simulink model "GP_CTC"  (R2019a)
settings: Solver=FixedStepAuto  StartTime=0  StopTime=300  FixedStep=0.005  RelTol=1e-3
model workspace: external: MAT-File (data not in the file)
libraries: RealTimeLearning x2, simulink x1
settings Model: SnapshotBufferSize=1  SnapshotInterval=1  Creator=aordonez  LastModifiedBy=alederer
settings SolverCC: AlgebraicLoopSolver=LineSearch
settings DataIOCC: SaveFormat=Array
settings DebuggingCC: PregeneratedLibrarySubsystemCodeDiagnostic=none  ArithmeticOperatorsInVariantConditions=warning
settings CodeAppCC: StateflowObjectComments=on

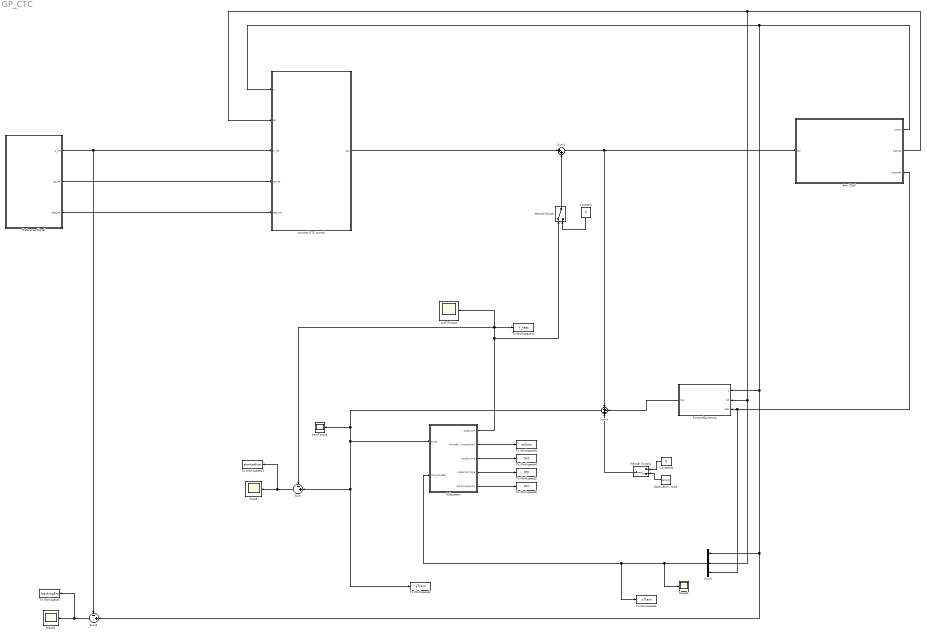
== system GP_CTC ==
  Arm 2DoF : Subsystem
  Constant : Constant  Value=0
  Constant1 : Constant  Value=0
  ForwardDynamics : MATLAB Function  TreatAsAtomicUnit=on
  Manual Switch : ManualSwitch
  Manual Switch1 : ManualSwitch  CurrentSetting=0
  Mux5 : Mux  Inputs=3
  Reference Signal : Subsystem
  Scope : Scope
  Scope1 : Scope
  Scope2 : Scope
  Subsystem : Subsystem
  Sum : Sum  Inputs=-+|
  Sum1 : Sum  Inputs=|++
  Sum2 : Sum  Inputs=-+|
  Sum5 : Sum  Inputs=+-+
  To Workspace1 : ToWorkspace  VariableName=xTrain  SampleTime=-1
      settings: Save2DSignal=2-D array (concatenate along first dimension)
  To Workspace10 : ToWorkspace  VariableName=Y_test  SampleTime=-1
      settings: Save2DSignal=2-D array (concatenate along first dimension)
  To Workspace11 : ToWorkspace  VariableName=absoluteError  SampleTime=-1
      settings: Save2DSignal=2-D array (concatenate along first dimension)
  To Workspace2 : ToWorkspace  VariableName=yTrain  SampleTime=-1
      settings: Save2DSignal=2-D array (concatenate along first dimension)
  To Workspace3 : ToWorkspace  VariableName=mNum  SampleTime=-1
      settings: Save2DSignal=2-D array (concatenate along first dimension)
  To Workspace4 : ToWorkspace  VariableName=tU0  SampleTime=-1
      settings: Save2DSignal=2-D array (concatenate along first dimension)
  To Workspace5 : ToWorkspace  VariableName=tP0  SampleTime=-1
      settings: Save2DSignal=2-D array (concatenate along first dimension)
  To Workspace6 : ToWorkspace  VariableName=pts  SampleTime=-1
      settings: Save2DSignal=2-D array (concatenate along first dimension)
  To Workspace7 : ToWorkspace  VariableName=trackingEror  SampleTime=-1
      settings: Save2DSignal=2-D array (concatenate along first dimension)
  nominal CTC control : Subsystem
  observation noise : RandomNumber  SampleTime=0.005
  outTrTorque : Scope
  trainTorque : Scope
  wires:
  Arm 2DoF/1(sigma) -> nominal CTC control/1(q), Sum2/2, Mux5/1, ForwardDynamics/1(q)
  Arm 2DoF/2(sigmad) -> nominal CTC control/2(dq), Mux5/2, ForwardDynamics/2(qd)
  Arm 2DoF/3(sigmadd) -> Mux5/3, ForwardDynamics/3(qdd)
  ForwardDynamics/1(tau) -> Sum5/2
  Sum/1 -> To Workspace11/1, Scope/1
  Mux5/1 -> Subsystem/2(p=[q,dq,ddq]), To Workspace1/1, Scope1/1
  Sum5/1 -> To Workspace2/1, Sum/2, Subsystem/1(e_tau), trainTorque/1
  Constant/1 -> Manual Switch/2
  Subsystem/1(prediction) -> Manual Switch/1, To Workspace10/1, Sum/1, outTrTorque/1
  Reference Signal/3(ddq_ref) -> nominal CTC control/5(ddq_ref)
  Reference Signal/2(dq_ref) -> nominal CTC control/4(dq_ref)
  Manual Switch/1 -> Sum1/2
  Sum1/1 -> Arm 2DoF/1(tau), Sum5/1
  Reference Signal/1(q_ref) -> nominal CTC control/3(q_ref), Sum2/1
  nominal CTC control/1(tau) -> Sum1/1
  Subsystem/2(#models in prediction) -> To Workspace3/1
  Subsystem/3(update time) -> To Workspace4/1
  Subsystem/4(prediction time) -> To Workspace5/1
  Subsystem/5(#training points) -> To Workspace6/1
  Constant1/1 -> Manual Switch1/1
  observation noise/1 -> Manual Switch1/2
  Manual Switch1/1 -> Sum5/3
  Sum2/1 -> To Workspace7/1, Scope2/1

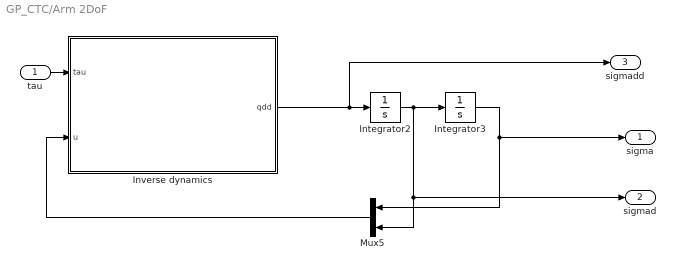
== system GP_CTC/Arm 2DoF ==
  tau : Inport
  Integrator2 : Integrator  InitialCondition=[0;0]
  Integrator3 : Integrator  InitialCondition=[0;0]
  Inverse dynamics : MATLAB Function  TreatAsAtomicUnit=on
  Mux5 : Mux  Inputs=2
  sigma : Outport
  sigmad : Outport  Port=2
  sigmadd : Outport  Port=3
  wires:
  Integrator3/1 -> sigma/1, Mux5/1
  tau/1 -> Inverse dynamics/1(tau)
  Integrator2/1 -> sigmad/1, Mux5/2, Integrator3/1
  Mux5/1 -> Inverse dynamics/2(u)
  Inverse dynamics/1(qdd) -> Integrator2/1, sigmadd/1

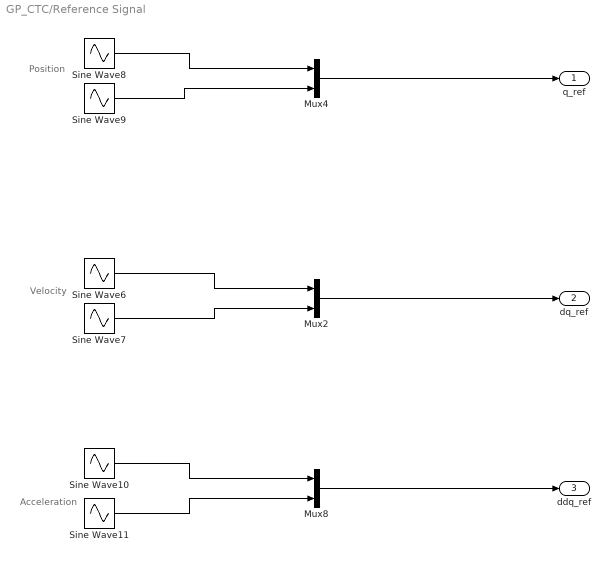
== system GP_CTC/Reference Signal ==
  note: Velocity
  note: Position
  note: Acceleration
  Mux2 : Mux  Inputs=2
  Mux4 : Mux  Inputs=2
  Mux8 : Mux  Inputs=2
  Sine Wave10 : Sin  Amplitude=-pi/6  Phase=pi/2  SampleTime=0
  Sine Wave11 : Sin  Amplitude=-pi/24  Frequency=0.5  Phase=pi/2  SampleTime=0
  Sine Wave6 : Sin  Amplitude=-pi/6  SampleTime=0
  Sine Wave7 : Sin  Amplitude=-pi/12  Frequency=0.5  SampleTime=0
  Sine Wave8 : Sin  Amplitude=pi/6  Phase=pi/2  SampleTime=0
  Sine Wave9 : Sin  Amplitude=pi/6  Frequency=0.5  Phase=pi/2  SampleTime=0
  q_ref : Outport
  dq_ref : Outport  Port=2
  ddq_ref : Outport  Port=3
  wires:
  Sine Wave10/1 -> Mux8/1
  Mux2/1 -> dq_ref/1
  Mux8/1 -> ddq_ref/1
  Mux4/1 -> q_ref/1
  Sine Wave8/1 -> Mux4/1
  Sine Wave11/1 -> Mux8/2
  Sine Wave6/1 -> Mux2/1
  Sine Wave9/1 -> Mux4/2
  Sine Wave7/1 -> Mux2/2

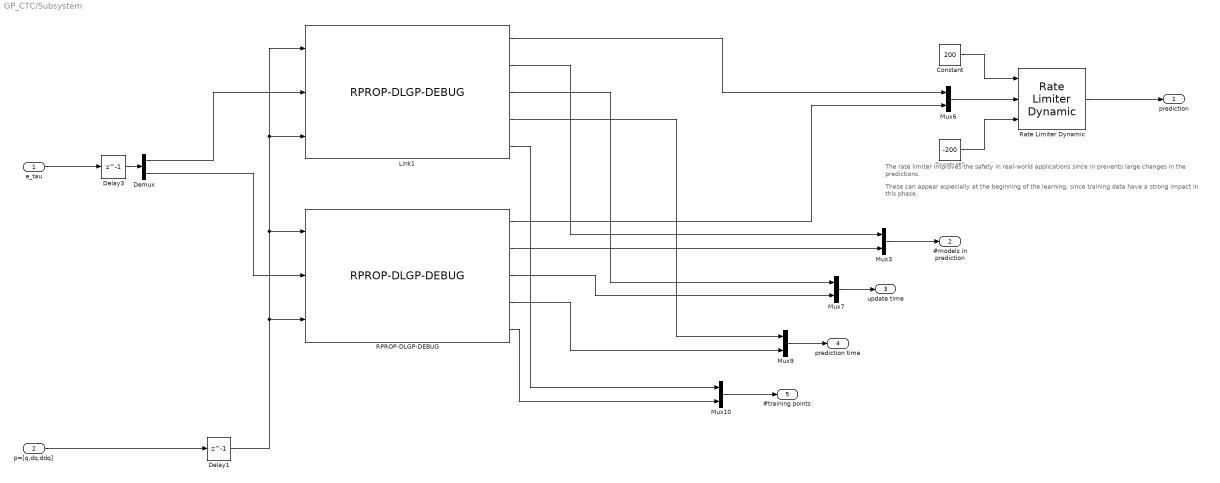
== system GP_CTC/Subsystem ==
  note: These can appear especially at the beginning of the learning, since training data have a strong impact in this phase.
  note: The rate limiter improves the safety in real-world applications since in prevents large changes in the predictions.
  e_tau : Inport
  p=[q,dq,ddq] : Inport  Port=2
  Constant : Constant  Value=200
  Constant1 : Constant  Value=-200
  Delay1 : Delay  DelayLength=1
  Delay3 : Delay  DelayLength=1
  Demux : Demux  Outputs=2
  Link1 : RealTimeLearning/RPROP-DLGP-DEBUG  ard=on  pts=50  N=10000  xSize=6  timeRate=0.005  divMethod=3  wo=300
      settings: SourceProductName=Real Time Learning
  Mux{3,6..7,9..10} (5 alike) : Mux  Inputs=2
  RPROP-DLGP-DEBUG : RealTimeLearning/RPROP-DLGP-DEBUG  ard=on  pts=50  N=10000  xSize=6  timeRate=0.005  divMethod=3  wo=300
      settings: SourceProductName=Real Time Learning
  Rate Limiter Dynamic : simulink/Discontinuities/Rate Limiter Dynamic
      settings: SourceProductName=Simulink
  prediction : Outport
  #models in prediction : Outport  Port=2
  update time : Outport  Port=3
  prediction time : Outport  Port=4
  #training points : Outport  Port=5
  wires:
  Delay3/1 -> Demux/1
  Link1/2 -> Mux3/1
  RPROP-DLGP-DEBUG/3 -> Mux7/2
  e_tau/1 -> Delay3/1
  RPROP-DLGP-DEBUG/2 -> Mux3/2
  Mux9/1 -> prediction time/1
  Demux/1 -> Link1/2
  Mux3/1 -> #models in prediction/1
  Link1/3 -> Mux7/1
  Link1/4 -> Mux9/1
  p=[q,dq,ddq]/1 -> Delay1/1
  Mux10/1 -> #training points/1
  Link1/5 -> Mux10/1
  Delay1/1 -> Link1/3, Link1/1, RPROP-DLGP-DEBUG/1, RPROP-DLGP-DEBUG/3
  Mux7/1 -> update time/1
  RPROP-DLGP-DEBUG/4 -> Mux9/2
  RPROP-DLGP-DEBUG/5 -> Mux10/2
  RPROP-DLGP-DEBUG/1 -> Mux6/2
  Demux/2 -> RPROP-DLGP-DEBUG/2
  Link1/1 -> Mux6/1
  Mux6/1 -> Rate Limiter Dynamic/2
  Constant/1 -> Rate Limiter Dynamic/1
  Constant1/1 -> Rate Limiter Dynamic/3
  Rate Limiter Dynamic/1 -> prediction/1

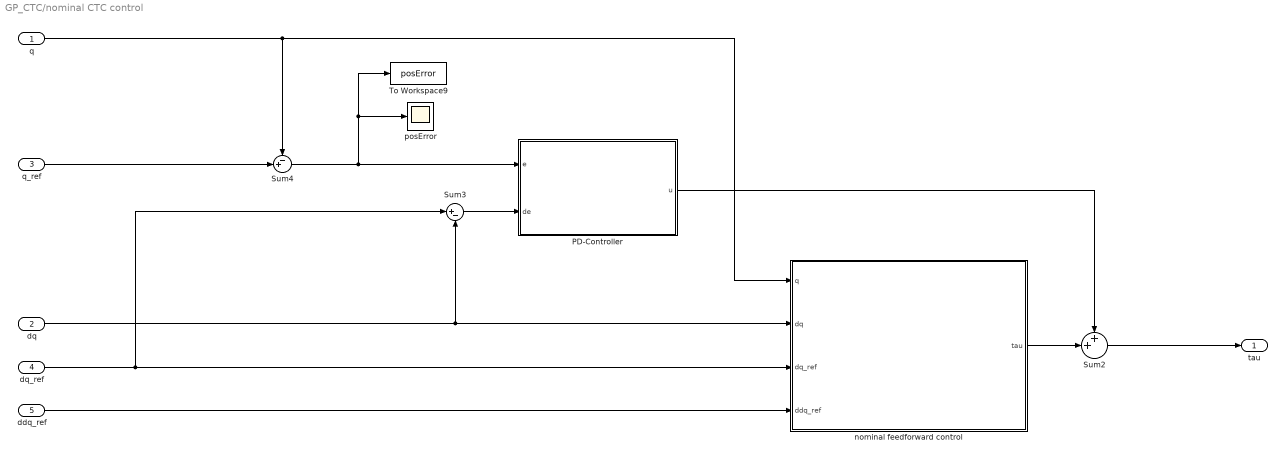
== system GP_CTC/nominal CTC control ==
  q : Inport
  dq : Inport  Port=2
  q_ref : Inport  Port=3
  dq_ref : Inport  Port=4
  ddq_ref : Inport  Port=5
  PD-Controller : Subsystem
  Sum2 : Sum  Inputs=++|
  Sum3 : Sum  Inputs=|+-
  Sum4 : Sum  Inputs=-+|
  To Workspace9 : ToWorkspace  VariableName=posError  SampleTime=-1
      settings: Save2DSignal=2-D array (concatenate along first dimension)
  nominal feedforward control : MATLAB Function  TreatAsAtomicUnit=on
  posError : Scope
  tau : Outport
  wires:
  q/1 -> nominal feedforward control/1(q), Sum4/1
  q_ref/1 -> Sum4/2
  ddq_ref/1 -> nominal feedforward control/4(ddq_ref)
  dq_ref/1 -> Sum3/1, nominal feedforward control/3(dq_ref)
  Sum4/1 -> To Workspace9/1, posError/1, PD-Controller/1(e)
  dq/1 -> Sum3/2, nominal feedforward control/2(dq)
  Sum2/1 -> tau/1
  PD-Controller/1(u) -> Sum2/1
  nominal feedforward control/1(tau) -> Sum2/2
  Sum3/1 -> PD-Controller/2(de)

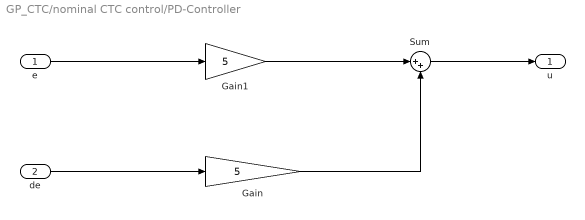
== system GP_CTC/nominal CTC control/PD-Controller ==
  e : Inport
  de : Inport  Port=2
  Gain : Gain  Gain=5
  Gain1 : Gain  Gain=5
  Sum : Sum  Inputs=|++
  u : Outport
  wires:
  e/1 -> Gain1/1
  de/1 -> Gain/1
  Gain1/1 -> Sum/1
  Gain/1 -> Sum/2
  Sum/1 -> u/1

== matlab function GP_CTC/ForwardDynamics ==
  data: q input; tau output; qd input; qdd input
function tau = CTcontrol(q,qd,qdd)
%{
inverse dynamics of a 2 DoF robotic arm

Inputs q: 2x1 vector. desired angular position
       qd: 2x1 vector. desired angular velocity
       qdd: 2x1 vector. desired angular acceleration

Output tau: 2x1 vector. Torques
%}
constant = 3.0;
Iz1 = constant;   %moment of inertia
Iz2 =constant;    
m1 = constant;    %mass
m2 = constant;
l1 = constant;    %length
l2 = constant;
r1 = l1;   %length to the center of mass
r2 = l2;
g = 9.81;  %gravity

a = Iz1 + Iz2 + m1*r1^2 + m2*( l1^2 + r2^2 );
b = m2*l1*r2;
d = Iz2 + m2*r2^2;

M = [ a + 2*b*cos( q(2) ),   d + b*cos( q(2) );
          d + b*cos( q(2) ),              d        ];

C = [ -b*sin( q(2) )*qd(2)     , -b*sin( q(2) )*( qd(1) + qd(2) );
       b*sin( q(2) )*qd(1)     ,               0                  ];

N = [ m1*g*r1*cos( q(1) ) + m2*g*( l1*cos( q(1) ) + r2*cos( q(1)+q(2) ) );
                    m2*g*r2*cos( q(1)+q(2) )                              ];
                
tau = M*(qdd) + C*(qd) +N;

== matlab function GP_CTC/nominal CTC control/nominal feedforward control ==
  data: q input; dq input; tau output; dq_ref input; ddq_ref input
function tau = CTcontrol(q,dq,dq_ref,ddq_ref)
%{
inverse dynamics of a 2 DoF robotic arm

Inputs q: 2x1 vector. given angular position
       qd: 2x1 vector. given angular velocity
       qdD: 2x1 vector. desired angular velocity 
       qddD: 2x1 vector. desired angular acceleration

Output tau: 2x1 vector. Torques
%}
constant = 3.0;
Iz1 = constant;   %moment of inertia
Iz2 =constant;    
m1 = constant;    %mass
m2 = constant;
l1 = constant;    %length
l2 = constant;
r1 = l1;   %length to the center of mass
r2 = l2;
g = 9.81;  %gravity

a = Iz1 + Iz2 + m1*r1^2 + m2*( l1^2 + r2^2 );
b = m2*l1*r2;
d = Iz2 + m2*r2^2;

M = [ a + 2*b*cos( q(2) ),   d + b*cos( q(2) );
          d + b*cos( q(2) ),              d        ];

C = [ -b*sin( q(2) )*dq(2)     , -b*sin( q(2) )*( dq(1) + dq(2) );
       b*sin( q(2) )*dq(1)     ,               0                  ];

N = [ m1*g*r1*cos( q(1) ) + m2*g*( l1*cos( q(1) ) + r2*cos( q(1)+q(2) ) );
                    m2*g*r2*cos( q(1)+q(2) )                              ];
                
tau = M*(ddq_ref) + C*(dq_ref) +N;

== matlab function GP_CTC/Arm 2DoF/Inverse dynamics ==
  data: tau input; u input; qdd output
function qdd = fcn(tau,u)
%{
inverse dynamics of a 2 DoF robotic arm
Inputs tau: 2x1 vector. Torques
       u: 4x1 vector [sigma1, sigma2, sigma1d, sigma2d]' position and speed
Output qdd: 2x1 vector with accelerations 
%}

Iz1 = 2;   %moment of inertia
Iz2 =2;    
m1 = 2;    %mass
m2 = 2;
l1 = 2;    %length
l2 = 2;
r1 = 2;   %length to the center of mass
r2 = 2;
g = 9.81;  %gravity

a = Iz1 + Iz2 + m1*r1^2 + m2*( l1^2 + r2^2 );
b = m2*l1*r2;
d = Iz2 + m2*r2^2;

M_inv = [ a + 2*b*cos( u(2) ),   d + b*cos( u(2) );
          d + b*cos( u(2) ),              d        ]^-1;

C = [ -b*sin( u(2) )*(2*u(3)*u(4) + u(4)^2); 
            b*sin( u(2) )*u(3)^2           ];
        

N = [ m1*g*r1*cos( u(1) ) + m2*g*( l1*cos( u(1) ) + r2*cos( u(1)+u(2) ) );
                    m2*g*r2*cos( u(1)+u(2) )                              ];

qdd = M_inv*( -C - N  + tau );
